simulink subsystem "CalibracionSensores"  (R2022b)
settings: Solver=VariableStepAuto  StartTime=0.0  StopTime=10.0  RelTol=1e-3
settings Model: Creator=Usuario  LastModifiedBy=Usuario

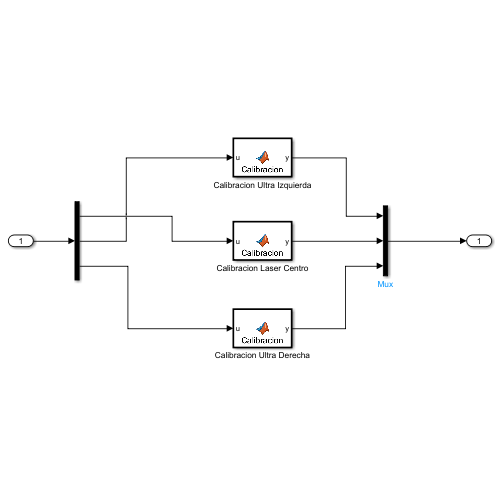
[thumbnail: Simulink's stored preview of the top-level diagram]
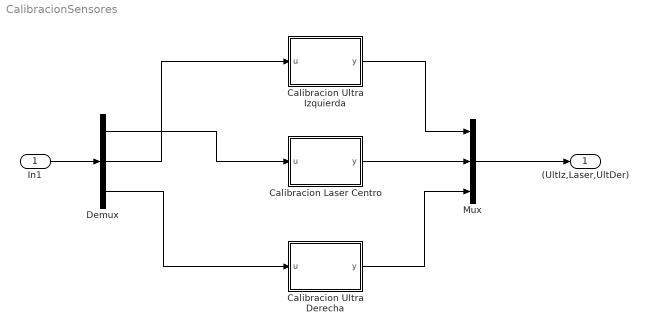
== system CalibracionSensores ==
  In1 : Inport
  Calibracion Laser Centro : MATLAB Function  TreatAsAtomicUnit=on
  Calibracion Ultra Derecha : MATLAB Function  TreatAsAtomicUnit=on
  Calibracion Ultra Izquierda : MATLAB Function  TreatAsAtomicUnit=on
  Demux : Demux  Outputs=3
  Mux : Mux  Inputs=3
  (UltIz,Laser,UltDer) : Outport
  wires:
  In1/1 -> Demux/1
  Demux/1 -> Calibracion Laser Centro/1(u)
  Demux/2 -> Calibracion Ultra Izquierda/1(u)
  Demux/3 -> Calibracion Ultra Derecha/1(u)
  Calibracion Laser Centro/1(y) -> Mux/2
  Calibracion Ultra Izquierda/1(y) -> Mux/1
  Calibracion Ultra Derecha/1(y) -> Mux/3
  Mux/1 -> (UltIz,Laser,UltDer)/1

== matlab function CalibracionSensores/Calibracion Ultra Izquierda ==
  data: u input; y output
function y = Calibracion(u)
a = 1.042894586;
b = 2.369184178;
c = a*u + b;
if c < 0
    c = 0;
end
y = c;

== matlab function CalibracionSensores/Calibracion Ultra Derecha ==
  data: u input; y output
function y = Calibracion(u)
a = 1.045647912;
b = 1.577328399;
c = a*u + b;
if c < 0
    c = 0;
end
y = c;

== matlab function CalibracionSensores/Calibracion Laser Centro ==
  data: u input; y output
function y = Calibracion(u)
a = 1.017824183;
b = -2.211652137;
c = a*u + b;
if c < 0
    c = 0;
end
y = c;
